simulink model "model_3_template"  (R2021b)
settings: Solver=FixedStepAuto  StartTime=0.0  StopTime=2  FixedStep=0.0005  RelTol=1e-3
undefined symbols (not defined in the file): A, BK, K, L, LC
settings Model: Creator=den  LastModifiedBy=den

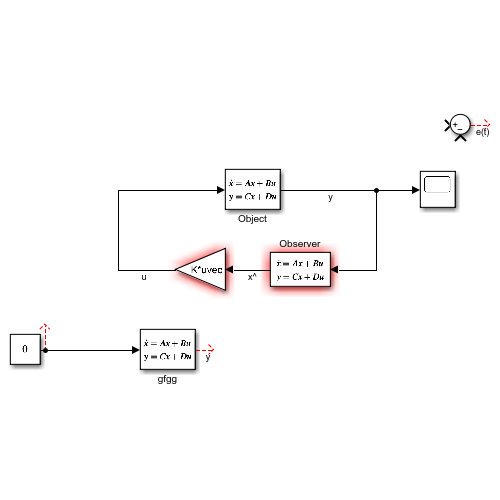
[thumbnail: Simulink's stored preview of the top-level diagram]
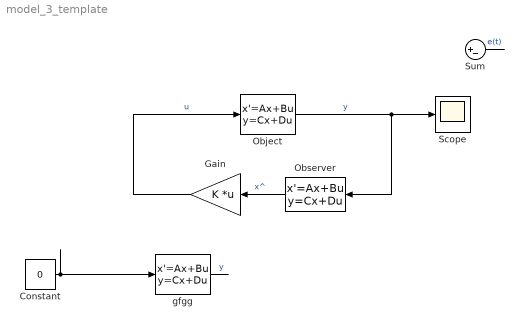
== system model_3_template ==
  Constant : Constant  Value=0
  Gain : Gain  Gain=K  Multiplication=Matrix(K*u) (u vector)
  Object : StateSpace  A=[5 -7 -5 1; -7 5 -1 5; -5 -1 5 7; 1 5 7 5]  B=[5; 7; 1; 9]  C=[0 0 2 2; 1 1 -1 1]  D=[0;0]  InitialCondition=0
  Observer : StateSpace  A=A+BK+LC  B=-L  C=[1 0 0 0; 0 1 0 0; 0 0 1 0; 0 0 0 1]  D=0  InitialCondition=0
  Scope : Scope
  Sum : Sum  Inputs=|+-
  gfgg : StateSpace  A=[0 5 0 0; -5 0 0 0; 0 0 0 1; 0 0 -1 0]  B=[0; 0; 0; 0]  C=[0 9 1 0]  D=0  InitialCondition=[1;1;1;1]
  wires:
  gfgg/1 -> ?  "y"
  Constant/1 -> gfgg/1
  Object/1 -> Scope/1, Observer/1  "y"
  Sum/1 -> ?  "e(t)"
  Observer/1 -> Gain/1  "x^"
  Gain/1 -> Object/1  "u"
